simulink subsystem "IMU"  (R2025b)
settings: Solver=VariableStepAuto  StartTime=0.0  StopTime=10.0  RelTol=1e-3
model mask{noise_accel=[1,1,1]*1e-3, bias_accel=[0 0 0], scale_accel=[1 0 0; 0 1 0; 0 0 1], lim_accel=inf, noise_gyro=[1,1,1]*1e-9, bias_gyro=[0 0 0], scale_gyro=[1 0 0; 0 1 0; 0 0 1], lim_gyro=inf, noise_mag=[1,1,1]*1e-2, bias_mag=[0 0 0], scale_mag=[1 0 0; 0 1 0; 0 0 1], limit_mag=0, noise_pres=0.2, bias_pres=0, scale_pres=1, limit_pres=[0, inf], Ssi=[1 0 0; 0 1 0; 0 0 1], Lsi=[0 0 0], lon=80.5204, lat=43.4643, year=2025}
  mask prompts: noise_accel "Accelerometer Noise Power"; bias_accel "Accelerometer Bias"; scale_accel "Accelerometer Scaling"; lim_accel "Accelerometer Limit"; noise_gyro "Gyro Noise Power"; bias_gyro "Gyro Bias"; scale_gyro "Gyro Scaling"; lim_gyro "Gyro Limit"; noise_mag "Mag Noise Power"; bias_mag "Mag Bias"; scale_mag "Mag Scaling"; limit_mag "Mag Limit"; noise_pres "Pressure Noise Power"; bias_pres "Pressure Bias"; scale_pres "Pressure Scaling"; limit_pres "Pressure Limit"; Ssi "Body to Sensor rotation"; Lsi "Sensor Location in Body frame"; lon "Geodetic Longitude (deg)"; lat "Geodetic Latitude (deg)"; year "Year (decimal)"
undefined symbols (not defined in the file): location, samplingrate
libraries: simulink x2, aerolibatmos2 x1, aerolibnav x1
settings Model: Creator=finnb  LastModifiedBy=trist

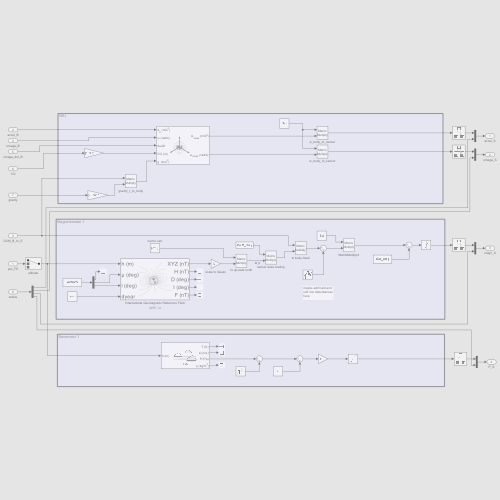
[thumbnail: Simulink's stored preview of the top-level diagram]
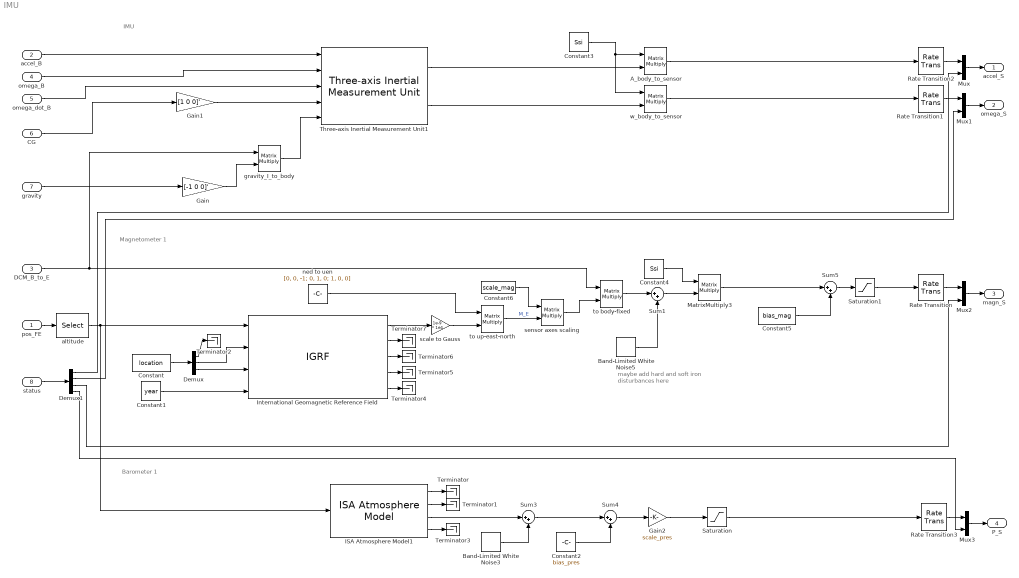
== system IMU ==
  note: Barometer 1
  note: Magnetometer 1
  note: IMU
  note: maybe add hard and soft iron disturbances here
  pos_FE : Inport
  accel_B : Inport  Port=2
  DCM_B_to_E : Inport  Port=3
  omega_B : Inport  Port=4
  omega_dot_B : Inport  Port=5
  CG : Inport  Port=6
  gravity : Inport  Port=7
  status : Inport  Port=8
  A_body_to_sensor : Product  Multiplication=Matrix(*)
  Band-Limited White Noise3 : simulink/Sources/Band-Limited White Noise  Cov=noise_pres  Ts=samplingrate  seed=[5781]
  Band-Limited White Noise5 : simulink/Sources/Band-Limited White Noise  Cov=noise_mag  Ts=samplingrate  seed=[298676]
  Constant : Constant  Value=location
  Constant1 : Constant  Value=year
  Constant2 : Constant  Value=bias_pres
  Constant3 : Constant  Value=Ssi
  Constant4 : Constant  Value=Ssi
  Constant5 : Constant  Value=bias_mag
  Constant6 : Constant  Value=scale_mag
  Demux : Demux  Outputs=3
  Demux1 : Demux
  Gain : Gain  Gain=[-1 0 0]'
  Gain1 : Gain  Gain=[1 0 0]'
  Gain2 : Gain  Gain=scale_pres
  ISA Atmosphere Model1 : aerolibatmos2/ISA Atmosphere Model  useExtended=on  action=Warning  custom=off  viscosityOut=off  g=9.80665  gamma=1.4  R=287.0531  L=0.0065  h_trop=11000  h_strat=20000  rho0=1.225  P0=101325  T0=288.15  h0=0  S=110.4  Tref=273.15  muref=1.716e-5
  International Geomagnetic Reference Field : IGRF  month=January  day=1  year=2020  sv_out=off
      settings: AttributesFormatString=%<generation>
  MatrixMultiply3 : Product  Multiplication=Matrix(*)
  Mux{,1..3} (4 alike) : Mux  Inputs=2
  Rate Transition{,1..3} (4 alike) : RateTransition  OutPortSampleTime=samplingrate
  Saturation : Saturate  UpperLimit=limit_pres(2)  LowerLimit=limit_pres(1)
  Saturation1 : Saturate  UpperLimit=limit_mag  LowerLimit=-limit_mag
  Sum{1,3..5} (4 alike) : Sum  Inputs=|++
  Terminator{,1..7} (8 alike) : Terminator
  Three-axis Inertial Measurement Unit1 : aerolibnav/Three-axis Inertial Measurement Unit  units=Metric (MKS)  imu=Lsi  i_Ts=samplingrate  dtype_a=off  w_a=190  z_a=0.707  a_sf_cc=scale_accel  a_bias=bias_accel  a_sat="[-lim_accel  -lim_accel  -lim_accel  lim_accel lim_accel lim_accel]"  dtype_g=off  w_g=190  z_g=0.707  g_sf_cc=scale_gyro  g_bias=bias_gyro  g_sens=[0 0 0]  g_sat="[-lim_gyro  -lim_gyro  -lim_gyro lim_gyro lim_gyro lim_gyro]"  i_rand=on  i_seeds=[23093 23094 23095 23096 23097 23098]  i_pow="[noise_accel,  noise_gyro]"
  altitude : Selector  InputPortWidth=3  IndexOptions=Index vector (dialog)  Indices=[1]  OutputSizes=1
  gravity_I_to_body : Product  Multiplication=Matrix(*)
  ned to uen : Constant  Value=[0, 0, -1; 0, 1, 0; 1, 0, 0]
  scale to Gauss : Gain  Gain=1e-9 * 1e4
  sensor axes scaling : Product  Multiplication=Matrix(*)
  to body-fixed : Product  Multiplication=Matrix(*)
  to up-east-north : Product  Multiplication=Matrix(*)
  w_body_to_sensor : Product  Multiplication=Matrix(*)
  accel_S : Outport  PortDimensions=4
  omega_S : Outport  Port=2  PortDimensions=4
  magn_S : Outport  Port=3  PortDimensions=4
  P_S : Outport  Port=4  PortDimensions=2
  wires:
  accel_B/1 -> Three-axis Inertial Measurement Unit1/1
  omega_B/1 -> Three-axis Inertial Measurement Unit1/2
  omega_dot_B/1 -> Three-axis Inertial Measurement Unit1/3
  CG/1 -> Gain1/1
  gravity_I_to_body/1 -> Three-axis Inertial Measurement Unit1/5
  Gain1/1 -> Three-axis Inertial Measurement Unit1/4
  Constant/1 -> Demux/1
  Demux/2 -> International Geomagnetic Reference Field/2
  International Geomagnetic Reference Field/1 -> scale to Gauss/1
  to up-east-north/1 -> sensor axes scaling/2  "M_E"
  Band-Limited White Noise5/1 -> Sum1/2
  Sum1/1 -> MatrixMultiply3/2
  A_body_to_sensor/1 -> Rate Transition2/1
  Constant3/1 -> w_body_to_sensor/1, A_body_to_sensor/1
  w_body_to_sensor/1 -> Rate Transition1/1
  Sum3/1 -> Sum4/1
  ISA Atmosphere Model1/3 -> Sum3/1
  Band-Limited White Noise3/1 -> Sum3/2
  Constant4/1 -> MatrixMultiply3/1
  Gain/1 -> gravity_I_to_body/2
  gravity/1 -> Gain/1
  Demux/3 -> International Geomagnetic Reference Field/3
  pos_FE/1 -> altitude/1
  Demux/1 -> Terminator2/1
  altitude/1 -> International Geomagnetic Reference Field/1, ISA Atmosphere Model1/1
  Constant1/1 -> International Geomagnetic Reference Field/4
  to body-fixed/1 -> Sum1/1
  ned to uen/1 -> to up-east-north/1
  scale to Gauss/1 -> to up-east-north/2
  DCM_B_to_E/1 -> gravity_I_to_body/1, to body-fixed/1
  Three-axis Inertial Measurement Unit1/1 -> A_body_to_sensor/2
  Three-axis Inertial Measurement Unit1/2 -> w_body_to_sensor/2
  ISA Atmosphere Model1/1 -> Terminator/1
  ISA Atmosphere Model1/2 -> Terminator1/1
  ISA Atmosphere Model1/4 -> Terminator3/1
  International Geomagnetic Reference Field/5 -> Terminator4/1
  International Geomagnetic Reference Field/4 -> Terminator5/1
  International Geomagnetic Reference Field/3 -> Terminator6/1
  International Geomagnetic Reference Field/2 -> Terminator7/1
  Sum4/1 -> Gain2/1
  Constant2/1 -> Sum4/2
  Gain2/1 -> Saturation/1
  MatrixMultiply3/1 -> Sum5/1
  Sum5/1 -> Saturation1/1
  Constant5/1 -> Sum5/2
  sensor axes scaling/1 -> to body-fixed/2
  Constant6/1 -> sensor axes scaling/1
  Saturation/1 -> Rate Transition3/1
  Saturation1/1 -> Rate Transition/1
  status/1 -> Demux1/1
  Rate Transition2/1 -> Mux/1
  Mux/1 -> accel_S/1
  Mux1/1 -> omega_S/1
  Rate Transition1/1 -> Mux1/1
  Demux1/2 -> Mux1/2
  Demux1/1 -> Mux/2
  Mux2/1 -> magn_S/1
  Rate Transition/1 -> Mux2/1
  Demux1/3 -> Mux2/2
  Mux3/1 -> P_S/1
  Rate Transition3/1 -> Mux3/1
  Demux1/4 -> Mux3/2
